simulink model "CommonModeSimulation"  (R2023a)
settings: Solver=FixedStepAuto  StartTime=0.0  StopTime=1/ffund  FixedStep=1e-8  RelTol=1e-3
InitFcn:
  | fsw=10e3;
  | ma=0.8;
  | ffund=100;
  | 
  | sym= pi/6;
settings Model: Creator=enesa  LastModifiedBy=enesa

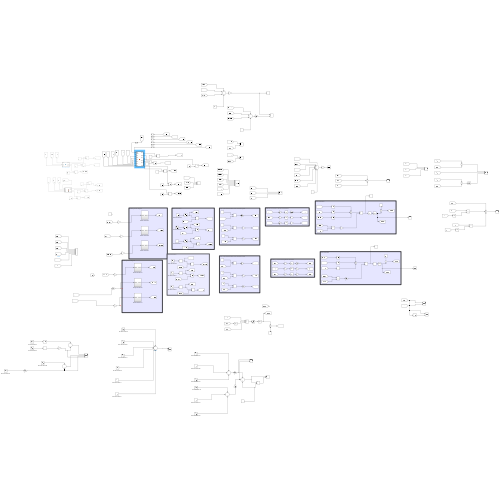
[thumbnail: Simulink's stored preview of the top-level diagram]
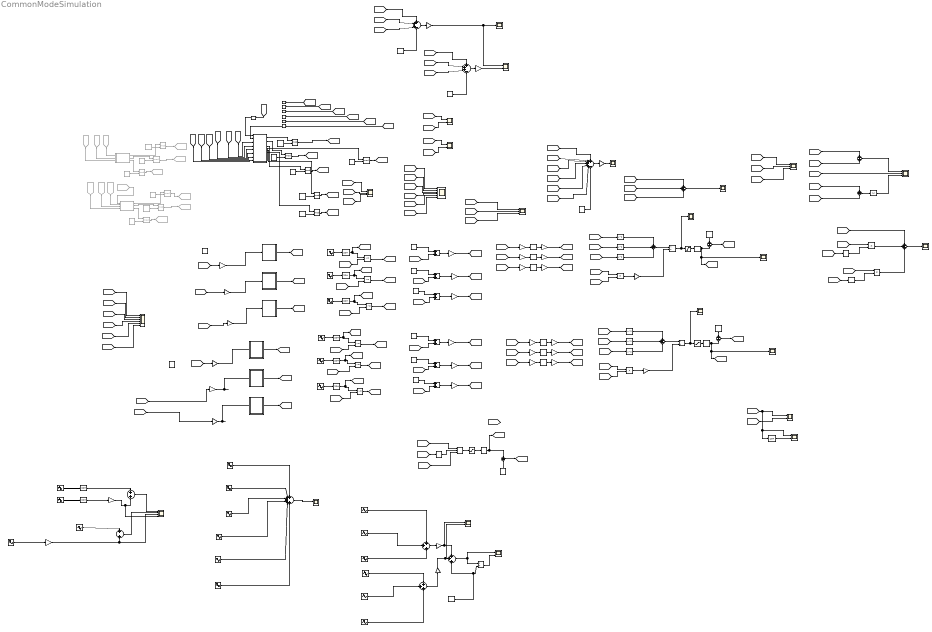
== system CommonModeSimulation ==
  note: Phi B calculation
  note: Switching component magnitude calculation
  note: Duty cycles determination from reference signals
  note: PWM Generation
  note: Creating Carrier Signals
  note: Creating Carrier Signals
  note: PWM Generation
  note: Duty cycles determination from reference signals
  note: Switching component magnitude calculation
  note: Phi B calculation
  Abs : Abs  SaturateOnIntegerOverflow=off
  Acos : Trigonometry  Operator=acos
  Acos1 : Trigonometry  Operator=acos
  Add{,1..5} (6 alike) : Sum
  Asin : Trigonometry  Operator=asin
  Constant : Constant  Value=-pi+pi/9
  Constant{1..2,9,15..17} (6 alike) : Constant  Commented=on  Value=2*pi
  Constant{3..5,10..12} (6 alike) : Constant
  Constant13 : Constant  Value=pi
  Constant14 : Constant  Value=0
  Constant18 : Constant  Value=3/2
  Constant19 : Constant  Value=3/2
  Constant{20..25} (6 alike) : Constant  Value=2*pi
  Constant26 : Constant  Value=3
  Constant6 : Constant  Value=3
  Constant7 : Constant  Value=pi
  Constant8 : Constant  Value=pi
  Cos : Trigonometry  Operator=cos
  Cos1 : Trigonometry  Operator=cos
  Delay{,1..6} (7 alike) : Delay  DelayLength=1  SampleTime=1/fsw
  Divide : Product  Inputs=*/
  Divide{1,3..4,6} (4 alike) : Product  Inputs=**
  Divide2 : Product  Inputs=**/
  Divide5 : Product  Inputs=*/
  Divide7 : Product  Inputs=*/
  From50 : From  Commented=on  GotoTag=DA
  From51 : From  Commented=on  GotoTag=DB
  From56 : From  Commented=on  GotoTag=DC
  From86 : From  Commented=on  GotoTag=DX
  From87 : From  Commented=on  GotoTag=DY
  From88 : From  Commented=on  GotoTag=DZ
  From96 : From  Commented=on  GotoTag=phiC2
  Gain{,1..2,17..19} (6 alike) : Gain  Gain=1/2
  Gain10 : Gain  Gain=2
  Gain{11..16} (6 alike) : Gain  Gain=-1
  Gain{4,6,8,20,22,24} (6 alike) : Gain  Gain=pi
  Gain{5,7,9,21,23,25} (6 alike) : Gain  Gain=2/pi
  Gain26 : Gain  Gain=2
  Gain27 : Gain  Gain=1/3
  Gain28 : Gain  Gain=1/3
  Gain{3,29..32} (5 alike) : Gain  Gain=1/6
  Goto19 : Goto  Commented=on  GotoTag=phiB2
  Goto20 : Goto  Commented=on  GotoTag=phiA2
  Goto21 : Goto  Commented=on  GotoTag=phiC2
  Goto39 : Goto  Commented=on  GotoTag=phiY2
  Goto40 : Goto  Commented=on  GotoTag=phiX2
  Goto41 : Goto  Commented=on  GotoTag=phiZ2
  MATLAB Function : MATLAB Function  Commented=on  TreatAsAtomicUnit=on
  MATLAB Function1 : MATLAB Function  Commented=on  TreatAsAtomicUnit=on
  MATLAB Function2 : MATLAB Function  TreatAsAtomicUnit=on
  Mod{,1..5} (6 alike) : Math  Commented=on  Operator=mod
  Mod{6..11} (6 alike) : Math  Operator=mod
  Relational Operator{,1..5} (6 alike) : RelationalOperator  OutDataTypeStr=boolean  RndMeth=Simplest  InputSameDT=off
  Saturation : Saturate  UpperLimit=1  LowerLimit=-1
  Saturation1 : Saturate  UpperLimit=1  LowerLimit=-1
  Saturation2 : Saturate  UpperLimit=1  LowerLimit=-1
  Scope{,3,8..9} (4 alike) : Scope  NumInputPorts=3
  Scope1 : Scope  NumInputPorts=6
  Scope{4,10,13..14,18..21} (8 alike) : Scope  NumInputPorts=2
  Scope{2,5..7,11,15..17} (8 alike) : Scope
  Scope12 : Scope  NumInputPorts=6
  Scope22 : Scope  NumInputPorts=4
  Sin{1..7} (7 alike) : Trigonometry
  Sine Wave-Phase A{,1,3,5} (4 alike) : Sin  Amplitude=ma  Frequency=2*pi*ffund  SampleTime=0
  Sine Wave-Phase A2 : Sin  Amplitude=ma  Frequency=2*pi*ffund*3  SampleTime=0
  Sine Wave-Phase A4 : Sin  Amplitude=ma  Frequency=2*pi*ffund*3  SampleTime=0
  Sine Wave-Phase A6 : Sin  Amplitude=ma  Frequency=2*pi*ffund*3  SampleTime=0
  Sine Wave-Phase B : Sin  Amplitude=ma  Frequency=2*pi*ffund  Phase=2*pi/3  SampleTime=0
  Sine Wave-Phase B1 : Sin  Amplitude=ma  Frequency=2*pi*ffund  Phase=2*pi/3  SampleTime=0
  Sine Wave-Phase B2 : Sin  Amplitude=ma  Frequency=2*pi*ffund*3  Phase=3*2*pi/3  SampleTime=0
  Sine Wave-Phase C : Sin  Amplitude=ma  Frequency=2*pi*ffund  Phase=-2*pi/3  SampleTime=0
  Sine Wave-Phase C1 : Sin  Amplitude=ma  Frequency=2*pi*ffund  Phase=-2*pi/3  SampleTime=0
  Sine Wave-Phase C2 : Sin  Amplitude=ma  Frequency=2*pi*ffund*3  Phase=-3*2*pi/3  SampleTime=0
  Sine Wave-Phase X : Sin  Amplitude=ma  Frequency=2*pi*ffund  Phase=sym  SampleTime=0
  Sine Wave-Phase X1 : Sin  Amplitude=ma  Frequency=2*pi*ffund  Phase=sym  SampleTime=0
  Sine Wave-Phase X2 : Sin  Amplitude=ma  Frequency=2*pi*ffund*3  Phase=sym*3  SampleTime=0
  Sine Wave-Phase Y : Sin  Amplitude=ma  Frequency=2*pi*ffund  Phase=2*pi/3+sym  SampleTime=0
  Sine Wave-Phase Y1 : Sin  Amplitude=ma  Frequency=2*pi*ffund  Phase=2*pi/3+sym  SampleTime=0
  Sine Wave-Phase Y2 : Sin  Amplitude=ma  Frequency=2*pi*ffund*3  Phase=(2*pi/3+sym)*3  SampleTime=0
  Sine Wave-Phase Z : Sin  Amplitude=ma  Frequency=2*pi*ffund  Phase=-2*pi/3+sym  SampleTime=0
  Sine Wave-Phase Z1 : Sin  Amplitude=ma  Frequency=2*pi*ffund  Phase=-2*pi/3+sym  SampleTime=0
  Sine Wave-Phase Z2 : Sin  Amplitude=ma  Frequency=2*pi*ffund*3  Phase=(-2*pi/3+sym)*3  SampleTime=0
  Square{1..6} (6 alike) : Math  Operator=square
  Sum : Sum  Inputs=++++++-
  Sum1 : Sum  Inputs=++-
  Sum10 : Sum  Inputs=++++++
  Sum{4,7,11..12,15} (5 alike) : Sum  Inputs=+++
  Sum13 : Sum  Inputs=+++-
  Sum14 : Sum  Inputs=+++-
  Sum16 : Sum
  Sum17 : Sum
  Sum{2..3,6,9} (4 alike) : Sum  Inputs=+-
  Sum5 : Sum
  Sum8 : Sum  Inputs=++-
  Triangle Generator-A : Subsystem
  Triangle Generator-A1 : Subsystem
  Triangle Generator-B : Subsystem
  Triangle Generator-B1 : Subsystem
  Triangle Generator-C : Subsystem
  Triangle Generator-C1 : Subsystem
  Zero-Order Hold : ZeroOrderHold  SampleTime=1/fsw
  Zero-Order Hold{6..8,12..14} (6 alike) : ZeroOrderHold  SampleTime=5/fsw
  Zero-Order Hold15 : ZeroOrderHold  SampleTime=1/ffund/40
  Zero-Order Hold2 : ZeroOrderHold  SampleTime=1/ffund/40
  wires:
  [CarrierA] -> Scope/1
  [CarrierB] -> Scope/2
  [CarrierC] -> Scope/3
  [PWMA] -> Scope1/1
  [PWMB] -> Scope1/2
  [PWMC] -> Scope1/3
  [PWMA] -> Sum/1
  [PWMB] -> Sum/2
  [PWMC] -> Sum/3
  Sum/1 -> Gain3/1
  Gain3/1 -> Scope2/1
  Constant6/1 -> Sum/7
  [DA] -> Scope3/1
  [DB] -> Scope3/2
  [DC] -> Scope3/3
  Triangle Generator-C/1(Carrier) -> [CarrierC]
  Triangle Generator-B/1(Carrier) -> [CarrierB]
  Triangle Generator-A/1(Carrier) -> [CarrierA]
  [CarrierB] -> Relational Operator1/2
  Relational Operator1/1 -> [PWMB]
  Relational Operator/1 -> [PWMA]
  Relational Operator2/1 -> [PWMC]
  [CarrierC] -> Relational Operator2/2
  Sine Wave-Phase A/1 -> Zero-Order Hold6/1
  Sine Wave-Phase C/1 -> Zero-Order Hold8/1
  [CarrierA] -> Relational Operator/2
  Sine Wave-Phase B/1 -> Zero-Order Hold7/1
  [sineC] -> Add2/2
  Constant4/1 -> Add1/1
  Constant3/1 -> Add/1
  Add2/1 -> Gain2/1
  Gain/1 -> [DA]
  Gain2/1 -> [DC]
  Add1/1 -> Gain1/1
  [sineB] -> Add1/2
  Constant5/1 -> Add2/1
  [sineA] -> Add/2
  Gain1/1 -> [DB]
  Add/1 -> Gain/1
  [DA] -> Gain4/1
  Sin1/1 -> Gain5/1
  Gain4/1 -> Sin1/1
  [DB] -> Gain6/1
  Gain7/1 -> [SBp]
  Sin3/1 -> Gain9/1
  Gain6/1 -> Sin2/1
  Gain8/1 -> Sin3/1
  [DC] -> Gain8/1
  Gain5/1 -> [SAp]
  Gain9/1 -> [SCp]
  Sin2/1 -> Gain7/1
  [SCp] -> Square3/1
  Acos/1 -> Sum2/2, Scope6/1, [alpha]
  Gain10/1 -> Divide/2
  Square3/1 -> Sum1/3
  [SAp] -> Divide1/1
  Sum1/1 -> Divide/1
  [SBp] -> Square1/1
  [SBp] -> Divide1/2
  Constant7/1 -> Sum2/1
  Divide/1 -> Scope5/1, Saturation/1
  Square2/1 -> Sum1/1
  [SAp] -> Square2/1
  Sum2/1 -> [phiB]
  Square1/1 -> Sum1/2
  Divide1/1 -> Gain10/1
  [alpha] -> Sin4/1
  [SBp] -> Divide2/1
  Sin4/1 -> Divide2/2
  [SCp] -> Divide2/3
  Divide2/1 -> Saturation1/1
  Asin/1 -> Sum3/1, [beta]
  Constant8/1 -> Sum3/2
  Sum3/1 -> [phic]
  [phiB] -> Scope10/1, Zero-Order Hold/1, Scope4/1
  [phic] -> Scope4/2
  [SBp] -> Divide3/1
  [phiB] -> Cos/1
  Cos/1 -> Divide3/2
  [phic] -> Cos1/1
  Cos1/1 -> Divide4/2
  [SCp] -> Divide4/1
  [SAp] -> Sum4/1
  Divide3/1 -> Sum4/2
  Divide4/1 -> Sum4/3
  Sum4/1 -> Scope7/1
  [SAp] -> Scope8/1
  [SBp] -> Scope8/2
  [SCp] -> Scope8/3
  [SAp] -> Sum5/1
  [SBp] -> Sum5/2
  Sum5/1 -> Scope9/1
  [SCp] -> Scope9/2
  [SAp] -> Sum6/1
  [SBp] -> Sum6/2
  Sum6/1 -> Abs/1
  Abs/1 -> Scope9/3
  Saturation/1 -> Acos/1
  Saturation1/1 -> Asin/1
  Zero-Order Hold/1 -> Scope10/2
  [DA] -> Sum7/1
  [DC] -> Sum7/3
  [DB] -> Sum7/2
  Sum7/1 -> Scope11/1
  [phiB2] -> Scope12/2
  [phiC2] -> Scope12/3
  From50/1 -> MATLAB Function/1(DA)
  From51/1 -> MATLAB Function/2(DB)
  From56/1 -> MATLAB Function/3(DC)
  [phiA2] -> Scope12/1
  [CarrierA] -> Scope13/1
  [PWMA] -> Scope13/2
  [CarrierA] -> Scope14/1
  [PWMB] -> Scope14/2
  Constant1/1 -> Mod/2
  Constant2/1 -> Mod1/2
  Constant9/1 -> Mod2/2
  Mod2/1 -> Goto19/1
  Mod/1 -> Goto21/1
  Mod1/1 -> Goto20/1
  MATLAB Function/1(phA) -> Mod1/1
  MATLAB Function/2(phB) -> Mod2/1
  MATLAB Function/3(phC) -> Mod/1
  [phiA2] -> Gain11/1
  [phiB2] -> Gain12/1
  [phiC2] -> Gain13/1
  Gain11/1 -> Triangle Generator-A/1(Phase)
  Gain13/1 -> Triangle Generator-C/1(Phase)
  Zero-Order Hold6/1 -> Relational Operator/1, [sineA]
  Zero-Order Hold7/1 -> [sineB], Relational Operator1/1
  Zero-Order Hold8/1 -> Relational Operator2/1, [sineC]
  Gain15/1 -> Triangle Generator-B1/1(Phase)
  Gain16/1 -> Triangle Generator-A1/1(Phase)
  Gain14/1 -> Triangle Generator-C1/1(Phase)
  Triangle Generator-C1/1(Carrier) -> [CarrierZ]
  Triangle Generator-A1/1(Carrier) -> [CarrierX]
  Triangle Generator-B1/1(Carrier) -> [CarrierY]
  Zero-Order Hold14/1 -> Relational Operator5/1, [sineZ]
  Zero-Order Hold13/1 -> [sineY], Relational Operator4/1
  Zero-Order Hold12/1 -> Relational Operator3/1, [sineX]
  Sine Wave-Phase Y/1 -> Zero-Order Hold13/1
  Relational Operator5/1 -> [PWMZ]
  [CarrierY] -> Relational Operator4/2
  Sine Wave-Phase Z/1 -> Zero-Order Hold14/1
  Relational Operator3/1 -> [PWMX]
  Sine Wave-Phase X/1 -> Zero-Order Hold12/1
  Relational Operator4/1 -> [PWMY]
  [CarrierZ] -> Relational Operator5/2
  [CarrierX] -> Relational Operator3/2
  [sineX] -> Add3/2
  [sineZ] -> Add5/2
  [sineY] -> Add4/2
  Constant11/1 -> Add4/1
  Add3/1 -> Gain17/1
  Gain19/1 -> [DZ]
  Add4/1 -> Gain18/1
  Constant12/1 -> Add5/1
  Add5/1 -> Gain19/1
  Constant10/1 -> Add3/1
  Gain18/1 -> [DY]
  Gain17/1 -> [DX]
  Gain23/1 -> [SYp]
  Sin6/1 -> Gain23/1
  Gain24/1 -> Sin7/1
  Gain25/1 -> [SZp]
  Sin7/1 -> Gain25/1
  [DY] -> Gain22/1
  Gain22/1 -> Sin6/1
  [DZ] -> Gain24/1
  Sin5/1 -> Gain21/1
  [DX] -> Gain20/1
  Gain21/1 -> [SXp]
  Gain20/1 -> Sin5/1
  [SXp] -> Divide6/1
  Square4/1 -> Sum8/2
  [SZp] -> Square6/1
  [SYp] -> Square4/1
  [SYp] -> Divide6/2
  Gain26/1 -> Divide5/2
  Square5/1 -> Sum8/1
  Divide6/1 -> Gain26/1
  Sum9/1 -> [phiY]
  [SXp] -> Square5/1
  Acos1/1 -> Sum9/2, Scope16/1, [alphaX]
  Divide5/1 -> Scope15/1, Saturation2/1
  Constant13/1 -> Sum9/1
  Square6/1 -> Sum8/3
  Sum8/1 -> Divide5/1
  Saturation2/1 -> Acos1/1
  [PWMX] -> Scope1/4
  [PWMY] -> Scope1/5
  [PWMZ] -> Scope1/6
  [PWMX] -> Sum/4
  [PWMZ] -> Sum/6
  [PWMY] -> Sum/5
  MATLAB Function1/1(phA) -> Mod4/1
  MATLAB Function1/3(phC) -> Mod3/1
  From87/1 -> MATLAB Function1/3(DB)
  Mod3/1 -> Goto41/1
  From86/1 -> MATLAB Function1/2(DA)
  Constant16/1 -> Mod4/2
  Mod5/1 -> Goto39/1
  Mod4/1 -> Goto40/1
  MATLAB Function1/2(phB) -> Mod5/1
  From88/1 -> MATLAB Function1/4(DC)
  Constant17/1 -> Mod5/2
  Constant15/1 -> Mod3/2
  [phiX2] -> Scope12/4
  [phiY2] -> Scope12/5
  [phiZ2] -> Scope12/6
  [phiY2] -> Gain15/1
  [phiZ2] -> Gain14/1
  Gain27/1 -> Scope18/1, Scope17/1
  [PWMA] -> Sum13/1
  Constant18/1 -> Sum13/4
  [PWMC] -> Sum13/3
  Sum13/1 -> Gain27/1
  [PWMB] -> Sum13/2
  [PWMY] -> Sum14/2
  Constant19/1 -> Sum14/4
  [PWMX] -> Sum14/1
  [PWMZ] -> Sum14/3
  Sum14/1 -> Gain28/1
  Gain28/1 -> Scope18/2
  From96/1 -> MATLAB Function1/1(ph)
  MATLAB Function2/1(phA) -> Mod7/1
  MATLAB Function2/3(phC) -> Mod6/1
  Mod6/1 -> [phiC2]
  Constant21/1 -> Mod7/2
  Mod8/1 -> [phiB2]
  Mod7/1 -> [phiA2]
  MATLAB Function2/2(phB) -> Mod8/1
  [DC] -> MATLAB Function2/5(DC)
  Constant22/1 -> Mod8/2
  Constant20/1 -> Mod6/2
  Mod9/1 -> [phiX2]
  MATLAB Function2/4(phX) -> Mod9/1
  Constant23/1 -> Mod9/2
  MATLAB Function2/5(phY) -> Mod10/1
  Constant24/1 -> Mod10/2
  Mod10/1 -> [phiY2]
  MATLAB Function2/6(phZ) -> Mod11/1
  Constant25/1 -> Mod11/2
  Mod11/1 -> [phiZ2]
  [phiX2] -> Gain16/1
  Sine Wave-Phase A1/1 -> Sum10/1
  Sine Wave-Phase B1/1 -> Sum10/2
  Sine Wave-Phase C1/1 -> Sum10/3
  Sine Wave-Phase X1/1 -> Sum10/4
  Sine Wave-Phase Y1/1 -> Sum10/5
  Sine Wave-Phase Z1/1 -> Sum10/6
  Sum10/1 -> Scope19/1
  Sine Wave-Phase B2/1 -> Sum11/2
  Sine Wave-Phase A2/1 -> Sum11/1
  Sine Wave-Phase C2/1 -> Sum11/3
  Sine Wave-Phase X2/1 -> Sum12/1
  Sine Wave-Phase Y2/1 -> Sum12/2
  Sine Wave-Phase Z2/1 -> Sum12/3
  Sum11/1 -> Gain29/1
  Sum12/1 -> Gain30/1
  Sum15/1 -> Scope20/1, Divide7/1
  Gain29/1 -> Scope21/1, Sum15/1
  Gain30/1 -> Scope21/2, Sum15/2
  Constant26/1 -> Sum15/3, Divide7/2
  Divide7/1 -> Scope20/2
  Sine Wave-Phase A4/1 -> Zero-Order Hold15/1
  Sine Wave-Phase A3/1 -> Zero-Order Hold2/1
  Gain31/1 -> Scope22/4, Sum16/2
  Sum16/1 -> Scope22/1
  Gain32/1 -> Scope22/3, Sum17/2
  Sine Wave-Phase A5/1 -> Sum17/1
  Sum17/1 -> Scope22/2
  Sine Wave-Phase A6/1 -> Gain32/1
  Zero-Order Hold2/1 -> Sum16/1
  Zero-Order Hold15/1 -> Gain31/1
  [DX] -> MATLAB Function2/6(DX)
  [DB] -> MATLAB Function2/4(DB)
  [DZ] -> MATLAB Function2/8(DZ)
  [DA] -> MATLAB Function2/3(DA)
  Gain12/1 -> Triangle Generator-B/1(Phase)
  [DY] -> MATLAB Function2/7(DY)
  Delay/1 -> MATLAB Function2/2(phZ1)
  [phiB2] -> Delay3/1
  [phiA2] -> Delay5/1
  [phiC2] -> Delay4/1
  [phiX2] -> Delay2/1
  [phiY2] -> Delay1/1
  [phiZ2] -> Delay/1
  Delay6/1 -> MATLAB Function2/1(DZ1)
  [DZ] -> Delay6/1

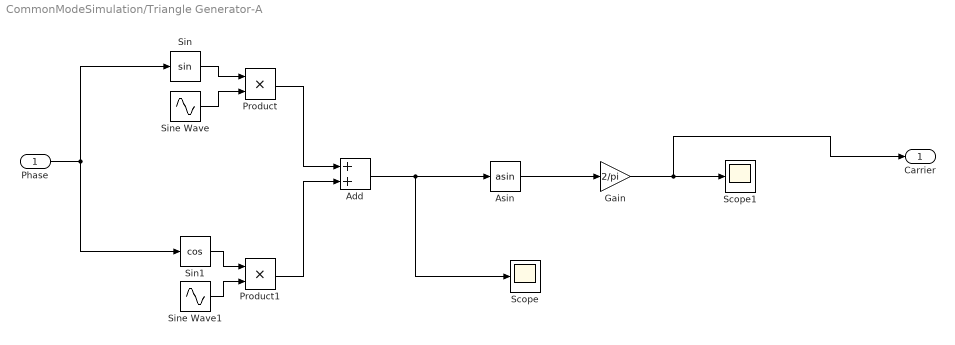
== system CommonModeSimulation/Triangle Generator-A ==
  Phase : Inport
  Add : Sum
  Asin : Trigonometry  Operator=asin
  Gain : Gain  Gain=2/pi
  Product : Product
  Product1 : Product
  Scope : Scope
  Scope1 : Scope
  Sin : Trigonometry
  Sin1 : Trigonometry  Operator=cos
  Sine Wave : Sin  Frequency=2*pi*fsw  SampleTime=0
  Sine Wave1 : Sin  Frequency=2*pi*fsw  Phase=-pi/2  SampleTime=0
  Carrier : Outport
  wires:
  Sin/1 -> Product/1
  Sine Wave/1 -> Product/2
  Phase/1 -> Sin1/1, Sin/1
  Product/1 -> Add/1
  Asin/1 -> Gain/1
  Gain/1 -> Carrier/1, Scope1/1
  Sine Wave1/1 -> Product1/2
  Product1/1 -> Add/2
  Add/1 -> Asin/1, Scope/1
  Sin1/1 -> Product1/1

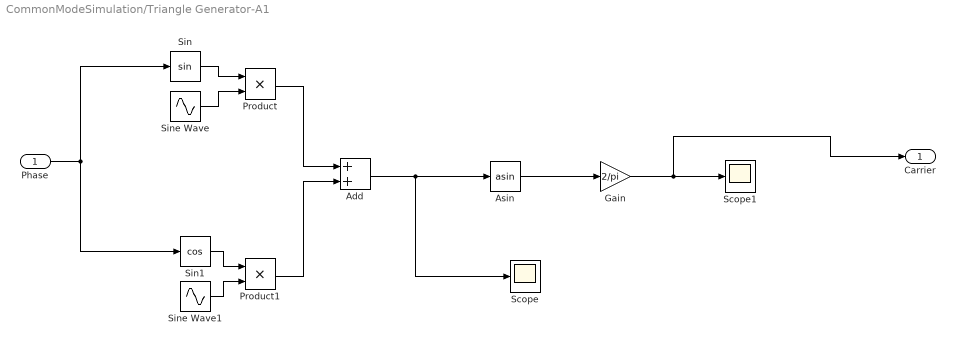
== system CommonModeSimulation/Triangle Generator-A1 ==
  Phase : Inport
  Add : Sum
  Asin : Trigonometry  Operator=asin
  Gain : Gain  Gain=2/pi
  Product : Product
  Product1 : Product
  Scope : Scope
  Scope1 : Scope
  Sin : Trigonometry
  Sin1 : Trigonometry  Operator=cos
  Sine Wave : Sin  Frequency=2*pi*fsw  SampleTime=0
  Sine Wave1 : Sin  Frequency=2*pi*fsw  Phase=-pi/2  SampleTime=0
  Carrier : Outport
  wires:
  Sin/1 -> Product/1
  Sine Wave/1 -> Product/2
  Phase/1 -> Sin1/1, Sin/1
  Product/1 -> Add/1
  Asin/1 -> Gain/1
  Gain/1 -> Carrier/1, Scope1/1
  Sine Wave1/1 -> Product1/2
  Product1/1 -> Add/2
  Add/1 -> Asin/1, Scope/1
  Sin1/1 -> Product1/1

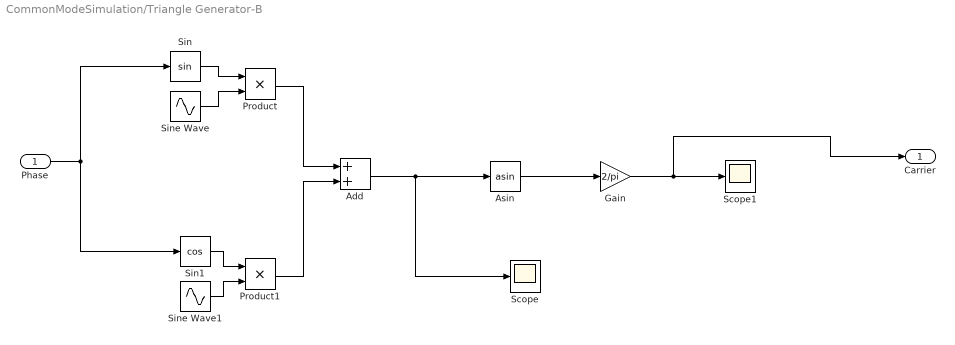
== system CommonModeSimulation/Triangle Generator-B ==
  Phase : Inport
  Add : Sum
  Asin : Trigonometry  Operator=asin
  Gain : Gain  Gain=2/pi
  Product : Product
  Product1 : Product
  Scope : Scope
  Scope1 : Scope
  Sin : Trigonometry
  Sin1 : Trigonometry  Operator=cos
  Sine Wave : Sin  Frequency=2*pi*fsw  SampleTime=0
  Sine Wave1 : Sin  Frequency=2*pi*fsw  Phase=-pi/2  SampleTime=0
  Carrier : Outport
  wires:
  Sin/1 -> Product/1
  Sine Wave/1 -> Product/2
  Phase/1 -> Sin1/1, Sin/1
  Product/1 -> Add/1
  Asin/1 -> Gain/1
  Gain/1 -> Carrier/1, Scope1/1
  Sine Wave1/1 -> Product1/2
  Product1/1 -> Add/2
  Add/1 -> Asin/1, Scope/1
  Sin1/1 -> Product1/1

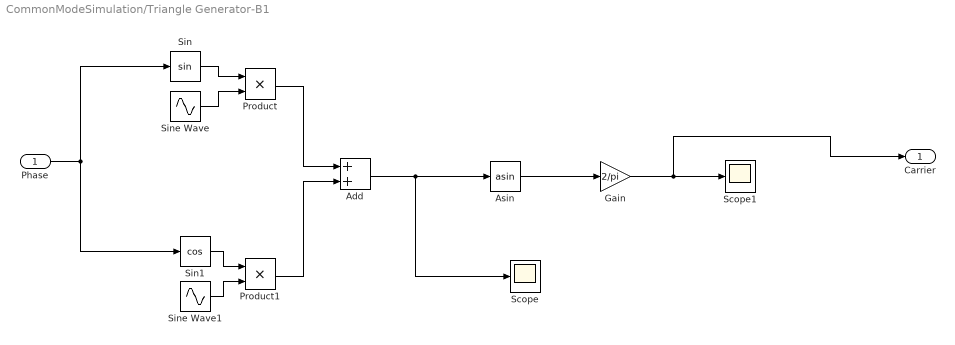
== system CommonModeSimulation/Triangle Generator-B1 ==
  Phase : Inport
  Add : Sum
  Asin : Trigonometry  Operator=asin
  Gain : Gain  Gain=2/pi
  Product : Product
  Product1 : Product
  Scope : Scope
  Scope1 : Scope
  Sin : Trigonometry
  Sin1 : Trigonometry  Operator=cos
  Sine Wave : Sin  Frequency=2*pi*fsw  SampleTime=0
  Sine Wave1 : Sin  Frequency=2*pi*fsw  Phase=-pi/2  SampleTime=0
  Carrier : Outport
  wires:
  Sin/1 -> Product/1
  Sine Wave/1 -> Product/2
  Phase/1 -> Sin1/1, Sin/1
  Product/1 -> Add/1
  Asin/1 -> Gain/1
  Gain/1 -> Carrier/1, Scope1/1
  Sine Wave1/1 -> Product1/2
  Product1/1 -> Add/2
  Add/1 -> Asin/1, Scope/1
  Sin1/1 -> Product1/1

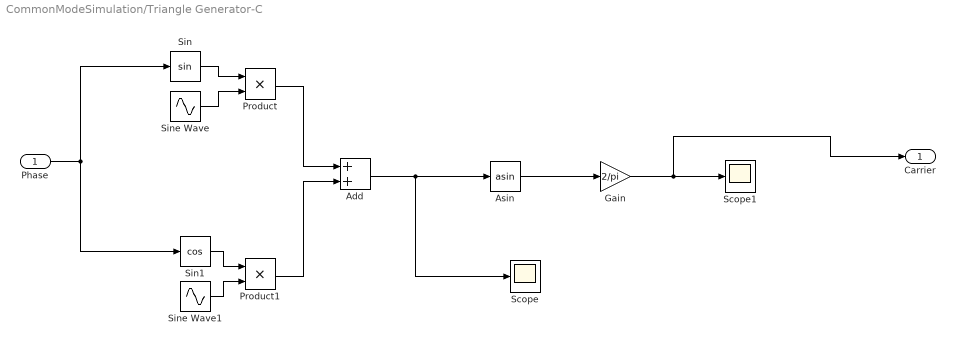
== system CommonModeSimulation/Triangle Generator-C ==
  Phase : Inport
  Add : Sum
  Asin : Trigonometry  Operator=asin
  Gain : Gain  Gain=2/pi
  Product : Product
  Product1 : Product
  Scope : Scope
  Scope1 : Scope
  Sin : Trigonometry
  Sin1 : Trigonometry  Operator=cos
  Sine Wave : Sin  Frequency=2*pi*fsw  SampleTime=0
  Sine Wave1 : Sin  Frequency=2*pi*fsw  Phase=-pi/2  SampleTime=0
  Carrier : Outport
  wires:
  Sin/1 -> Product/1
  Sine Wave/1 -> Product/2
  Phase/1 -> Sin1/1, Sin/1
  Product/1 -> Add/1
  Asin/1 -> Gain/1
  Gain/1 -> Carrier/1, Scope1/1
  Sine Wave1/1 -> Product1/2
  Product1/1 -> Add/2
  Add/1 -> Asin/1, Scope/1
  Sin1/1 -> Product1/1

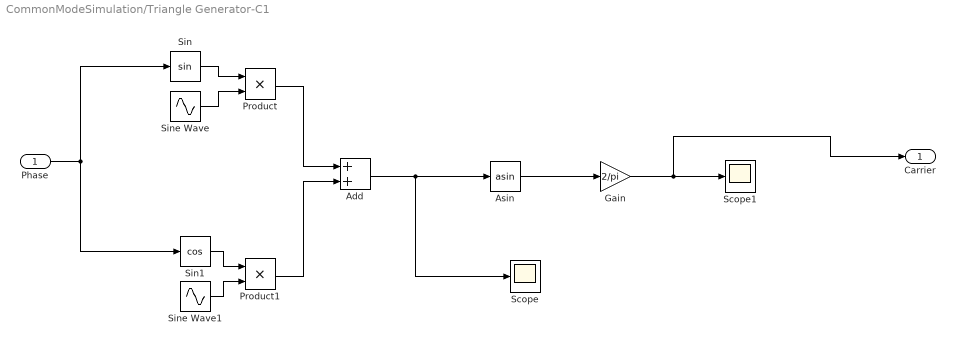
== system CommonModeSimulation/Triangle Generator-C1 ==
  Phase : Inport
  Add : Sum
  Asin : Trigonometry  Operator=asin
  Gain : Gain  Gain=2/pi
  Product : Product
  Product1 : Product
  Scope : Scope
  Scope1 : Scope
  Sin : Trigonometry
  Sin1 : Trigonometry  Operator=cos
  Sine Wave : Sin  Frequency=2*pi*fsw  SampleTime=0
  Sine Wave1 : Sin  Frequency=2*pi*fsw  Phase=-pi/2  SampleTime=0
  Carrier : Outport
  wires:
  Sin/1 -> Product/1
  Sine Wave/1 -> Product/2
  Phase/1 -> Sin1/1, Sin/1
  Product/1 -> Add/1
  Asin/1 -> Gain/1
  Gain/1 -> Carrier/1, Scope1/1
  Sine Wave1/1 -> Product1/2
  Product1/1 -> Add/2
  Add/1 -> Asin/1, Scope/1
  Sin1/1 -> Product1/1

== matlab function CommonModeSimulation/MATLAB Function1 ==
  data: ph input; DA input; phA output; DB input; DC input; phB output; phC output
function [phA, phB,phC] = fcn(ph, DA,DB,DC)
phA=0;
phB=((DA+DB)/2)*2*pi;
phC= (((DA+DC)/2)+DB)*2*pi;


end

== matlab function CommonModeSimulation/MATLAB Function ==
  data: DA input; phA output; DB input; DC input; phB output; phC output
function [phA, phB,phC] = fcn(DA,DB,DC)
phA=0;
phB=((DA+DB)/2)*2*pi;
phC= (((DA+DC)/2)+DB)*2*pi;


end

== matlab function CommonModeSimulation/MATLAB Function2 ==
  data: DZ1 input; phZ1 input; DA input; phA output; DB input; DC input; phB output; phC output; DX input; DY input; DZ input; phX output; phY output; phZ output
function [phA, phB,phC,phX,phY,phZ] = fcn(DZ1,phZ1, DA,DB,DC, DX, DY, DZ)

phA= phZ1+(DA+DZ1)*pi;
phB= phA+ (DA+DB)*pi;
phC= phB+ (DB+DC)*pi;
phX=phC+ (DX+DC)*pi;
phY= phX+ (DX+DY)*pi;
phZ= phY+ (DZ+DY)*pi;


% phA= 0;
% phB=((DA+DB)/2)*2*pi;
% phC= (((DA+DC)/2)+DB)*2*pi;
% phX= (((DA+DX)/2)+DB+DC)*2*pi;
% phY= (((DA+DY)/2)+DB+DC+DX)*2*pi;
% phZ= (((DA+DZ)/2)+DB+DC+DX+DY)*2*pi;


end
